simulink model "supply_ship_mdl"  (Simulink 8.9)
settings: Solver=ode1  StartTime=0  StopTime=300  FixedStep=delta_t  RelTol=1e-3  EnableMultiTasking=on
values from neighbouring files (symbols this model uses):
  K1 = B(1,1)/M(1,1)    [init.m]
  K2 = (M(2,2)*B(3,2)-M(2,3)*B(2,2))/(M(2,2)*M(3,3)-M(2,3)*M(2,3))    [init.m]
  psi0 = 0    [init.m]
  r0 = 0    [init.m]
  u0 = 0    [init.m]
  v0 = 0    [init.m]
  x0 = -200    [init.m]
  y0 = 200    [init.m]
settings Model: Creator=frk_moe  LastModifiedBy=signemoe
settings OptimizationCC: ExpressionDepthLimit=2147483647
settings DebuggingCC: SolverPrmCheckMsg=warning

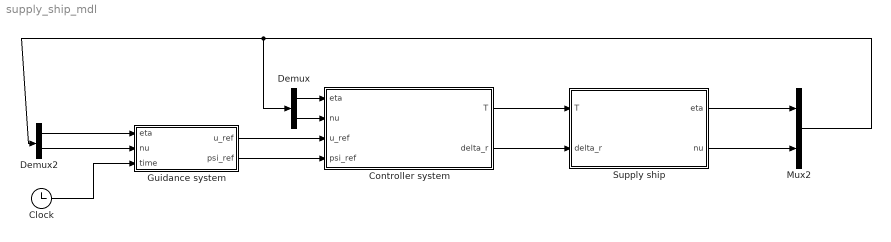
== system supply_ship_mdl ==
  Clock : Clock
  Controller system : Subsystem
  Demux : Demux  Outputs=2
  Demux2 : Demux  Outputs=2
  Guidance system : Subsystem
  Mux2 : Mux  Inputs=2
  Supply ship : Subsystem
  wires:
  Controller system/1(T) -> Supply ship/1(T)
  Supply ship/1(eta) -> Mux2/1
  Supply ship/2(nu) -> Mux2/2
  Mux2/1 -> Demux2/1, Demux/1
  Demux/2 -> Controller system/2(nu)
  Guidance system/2(psi_ref) -> Controller system/4(psi_ref)
  Guidance system/1(u_ref) -> Controller system/3(u_ref)
  Demux2/1 -> Guidance system/1(eta)
  Demux2/2 -> Guidance system/2(nu)
  Clock/1 -> Guidance system/3(time)
  Demux/1 -> Controller system/1(eta)
  Controller system/2(delta_r) -> Supply ship/2(delta_r)

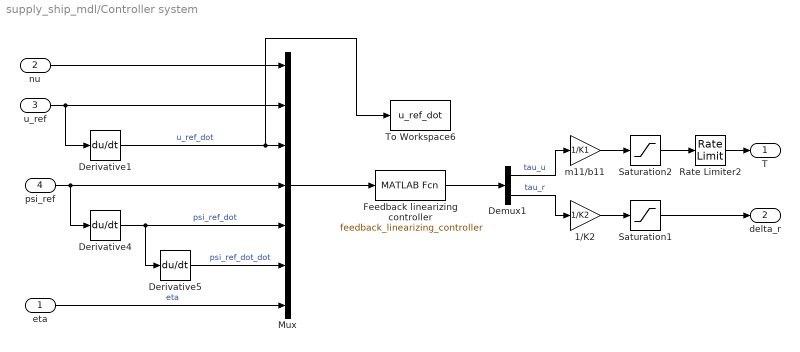
== system supply_ship_mdl/Controller system ==
  eta : Inport
  nu : Inport  Port=2
  u_ref : Inport  Port=3
  psi_ref : Inport  Port=4
  1/K2 : Gain  Gain=1/K2
  Demux1 : Demux  Outputs=2
  Derivative1 : Derivative
  Derivative4 : Derivative
  Derivative5 : Derivative
  Feedback linearizing controller : MATLABFcn  MATLABFcn=feedback_linearizing_controller  OutputDimensions=2
  Mux : Mux  Inputs=7
  Rate Limiter2 : RateLimiter  RisingSlewLimit=500000  FallingSlewLimit=-500000  SampleTimeMode=inherited
  Saturation1 : Saturate  UpperLimit=pi/2  LowerLimit=-pi/2
  Saturation2 : Saturate  UpperLimit=100000000  LowerLimit=-100000000
  To Workspace6 : ToWorkspace  VariableName=u_ref_dot  SaveFormat=Structure With Time  SampleTime=-1
  m11/b11 : Gain  Gain=1/K1
  T : Outport
  delta_r : Outport  Port=2
  wires:
  Mux/1 -> Feedback linearizing controller/1
  u_ref/1 -> Derivative1/1, Mux/2
  Derivative1/1 -> To Workspace6/1, Mux/3  "u_ref_dot"
  nu/1 -> Mux/1
  Feedback linearizing controller/1 -> Demux1/1
  Demux1/1 -> m11/b11/1  "tau_u"
  Demux1/2 -> 1/K2/1  "tau_r"
  eta/1 -> Mux/7  "eta"
  psi_ref/1 -> Mux/4, Derivative4/1
  Derivative4/1 -> Mux/5, Derivative5/1  "psi_ref_dot"
  Derivative5/1 -> Mux/6  "psi_ref_dot_dot"
  1/K2/1 -> Saturation1/1
  Saturation2/1 -> Rate Limiter2/1
  Rate Limiter2/1 -> T/1
  m11/b11/1 -> Saturation2/1
  Saturation1/1 -> delta_r/1

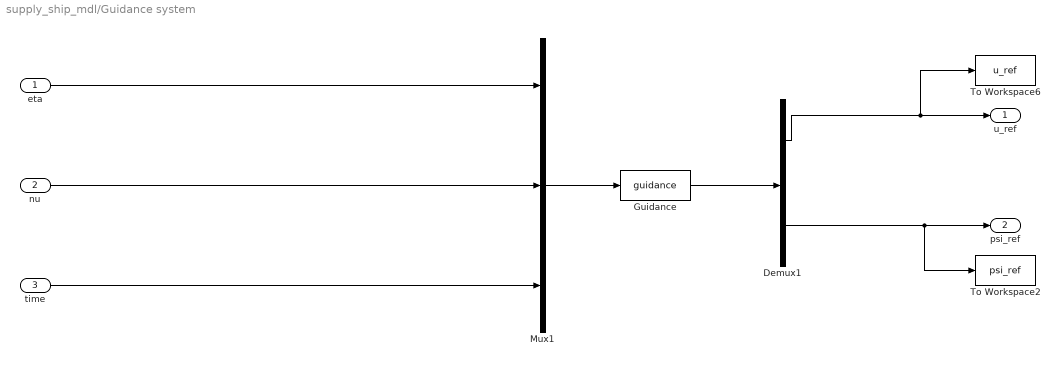
== system supply_ship_mdl/Guidance system ==
  eta : Inport
  nu : Inport  Port=2
  time : Inport  Port=3
  Demux1 : Demux  Outputs=2
  Guidance : MATLABFcn  MATLABFcn=guidance  OutputDimensions=2
  Mux1 : Mux  Inputs=3
  To Workspace2 : ToWorkspace  VariableName=psi_ref  SaveFormat=Structure With Time  SampleTime=-1
  To Workspace6 : ToWorkspace  VariableName=u_ref  SaveFormat=Structure With Time  SampleTime=-1
  u_ref : Outport
  psi_ref : Outport  Port=2
  wires:
  Guidance/1 -> Demux1/1
  Demux1/1 -> To Workspace6/1, u_ref/1
  Demux1/2 -> psi_ref/1, To Workspace2/1
  Mux1/1 -> Guidance/1
  eta/1 -> Mux1/1
  nu/1 -> Mux1/2
  time/1 -> Mux1/3

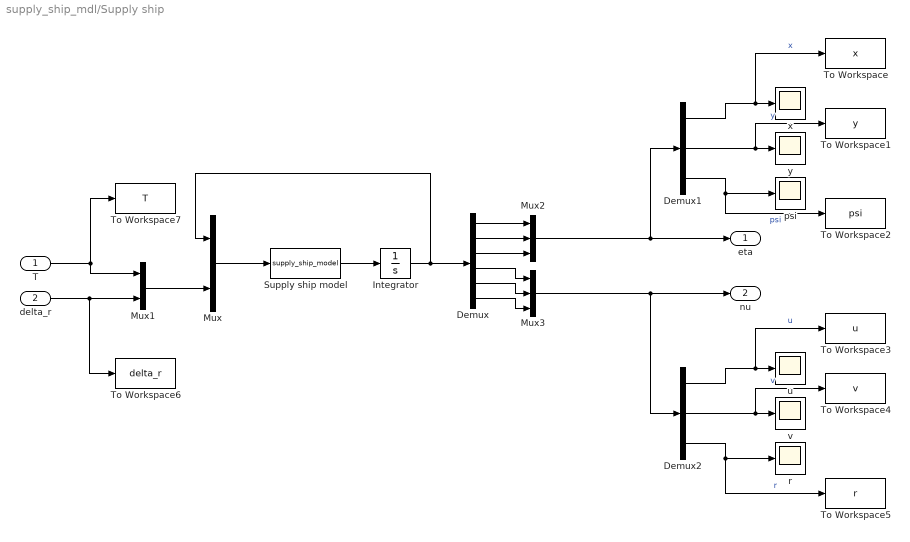
== system supply_ship_mdl/Supply ship ==
  T : Inport
  delta_r : Inport  Port=2
  Demux : Demux  Outputs=6
  Demux1 : Demux  Outputs=3
  Demux2 : Demux  Outputs=3
  Integrator : Integrator  InitialCondition=[x0;y0;psi0;u0;v0;r0]
  Mux : Mux  Inputs=2
  Mux1 : Mux  Inputs=2
  Mux2 : Mux  Inputs=3
  Mux3 : Mux  Inputs=3
  Supply ship model : MATLABFcn  MATLABFcn=supply_ship_model  OutputDimensions=6
  To Workspace : ToWorkspace  VariableName=x  SaveFormat=Structure With Time  SampleTime=-1
  To Workspace1 : ToWorkspace  VariableName=y  SaveFormat=Structure With Time  SampleTime=-1
  To Workspace2 : ToWorkspace  VariableName=psi  SaveFormat=Structure With Time  SampleTime=-1
  To Workspace3 : ToWorkspace  VariableName=u  SaveFormat=Structure With Time  SampleTime=-1
  To Workspace4 : ToWorkspace  VariableName=v  SaveFormat=Structure With Time  SampleTime=-1
  To Workspace5 : ToWorkspace  VariableName=r  SaveFormat=Structure With Time  SampleTime=-1
  To Workspace6 : ToWorkspace  VariableName=delta_r  SaveFormat=Structure With Time  SampleTime=-1
  To Workspace7 : ToWorkspace  VariableName=T  SaveFormat=Structure With Time  SampleTime=-1
  psi : Scope
  r : Scope
  u : Scope
  v : Scope
  x : Scope
  y : Scope
  eta : Outport
  nu : Outport  Port=2
  wires:
  Mux/1 -> Supply ship model/1
  Mux1/1 -> Mux/2
  Supply ship model/1 -> Integrator/1
  Integrator/1 -> Demux/1, Mux/1
  Demux/1 -> Mux2/1
  Demux/2 -> Mux2/2
  Demux/3 -> Mux2/3
  Demux/4 -> Mux3/1
  Demux/5 -> Mux3/2
  Demux/6 -> Mux3/3
  Mux2/1 -> eta/1, Demux1/1
  Mux3/1 -> nu/1, Demux2/1
  Demux1/1 -> x/1, To Workspace/1  "x"
  Demux1/2 -> y/1, To Workspace1/1  "y"
  Demux1/3 -> psi/1, To Workspace2/1  "psi"
  Demux2/1 -> u/1, To Workspace3/1  "u"
  Demux2/2 -> v/1, To Workspace4/1  "v"
  Demux2/3 -> r/1, To Workspace5/1  "r"
  delta_r/1 -> To Workspace6/1, Mux1/2
  T/1 -> To Workspace7/1, Mux1/1
